simulink model "Digitizing_3delays_1us_wNodes"  (R2014a)
settings: Solver=FixedStepDiscrete  StartTime=0.0  StopTime=0.0  FixedStep=1  RelTol=1e-3
undefined symbols (not defined in the file): inputPulse
libraries: opticalComponentLibrary x22
settings Model: Creator=Nithya Menon  LastModifiedBy=Alexander

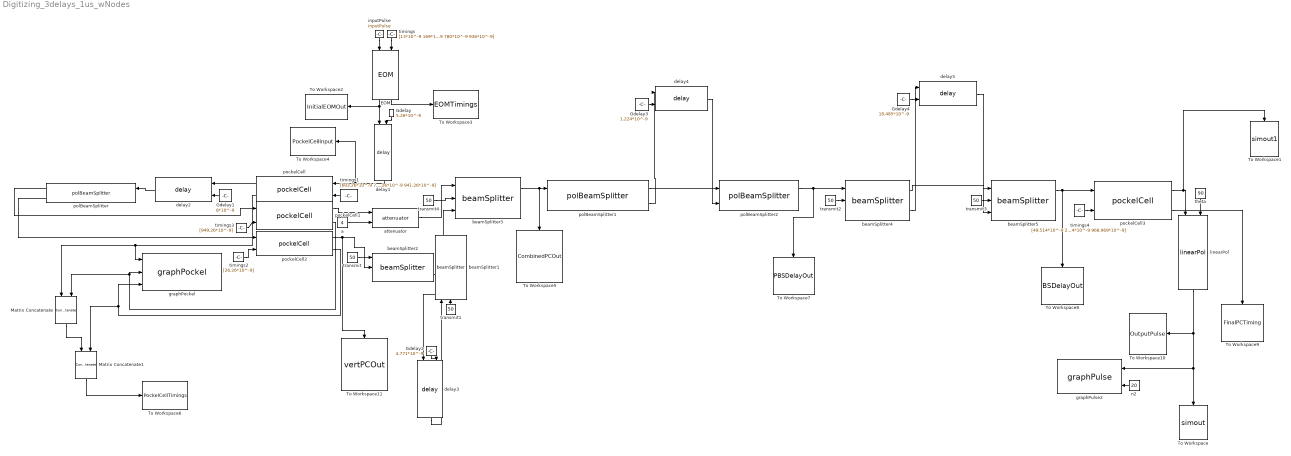
== system Digitizing_3delays_1us_wNodes ==
  EOM : opticalComponentLibrary/EOM
  Gdelay : Constant  Value=5.26*10^-9
  Gdelay1 : Constant  Value=8*10^-9
  Gdelay2 : Constant  Value=4.771*10^-9
  Gdelay3 : Constant  Value=1.224*10^-9
  Gdelay4 : Constant  Value=18.485*10^-9
  Matrix Concatenate : Concatenate  Mode=Multidimensional array  ConcatenateDimension=2
  Matrix Concatenate1 : Concatenate  Mode=Multidimensional array  ConcatenateDimension=2
  To Workspace : ToWorkspace  VariableName=simout  SampleTime=-1
  To Workspace1 : ToWorkspace  VariableName=simout1  SampleTime=-1
  To Workspace10 : ToWorkspace  VariableName=OutputPulse  SampleTime=-1
  To Workspace11 : ToWorkspace  VariableName=vertPCOut  SampleTime=-1
  To Workspace2 : ToWorkspace  VariableName=InitialEOMOut  SampleTime=-1
  To Workspace3 : ToWorkspace  VariableName=EOMTimings  SampleTime=-1
  To Workspace4 : ToWorkspace  VariableName=PockelCellInput  SampleTime=-1
  To Workspace5 : ToWorkspace  VariableName=CombinedPCOut  SampleTime=-1
  To Workspace6 : ToWorkspace  VariableName=PockelCellTimings  SampleTime=-1
  To Workspace7 : ToWorkspace  VariableName=PBSDelayOut  SampleTime=-1
  To Workspace8 : ToWorkspace  VariableName=BSDelayOut  SampleTime=-1
  To Workspace9 : ToWorkspace  VariableName=FinalPCTiming  SampleTime=-1
  a : Constant  Value=4
  attenuator : opticalComponentLibrary/attenuator
  beamSplitter{1..5} (5 alike) : opticalComponentLibrary/beamSplitter
  delay{1..5} (5 alike) : opticalComponentLibrary/delay
  graphPockel : opticalComponentLibrary/graphPockel
  graphPulse2 : opticalComponentLibrary/graphPulse
  inputPulse : Constant  Value=inputPulse
  linearPol : opticalComponentLibrary/linearPol
  n2 : Constant  Value=20
  pockelCell{,1..3} (4 alike) : opticalComponentLibrary/pockelCell
  polBeamSplitter : opticalComponentLibrary/polBeamSplitter
  polBeamSplitter1 : opticalComponentLibrary/polBeamSplitter
  polBeamSplitter2 : opticalComponentLibrary/polBeamSplitter
  theta : Constant  Value=90
  timings : Constant  Value="[13*10^-9 169*10^-9 351*10^-9  598*10^-9 780*10^-9 936*10^-9]"
  timings1 : Constant  Value=[603.26*10^-9 783.26*10^-9 941.26*10^-9]
  timings2 : Constant  Value=[26.26*10^-9]
  timings3 : Constant  Value=[949.26*10^-9]
  timings4 : Constant  Value=[49.514*10^-9 206.739*10^-9 370.254*10^-9 611.26*10^-9 811.744*10^-9 968.969*10^-9]
  transmit{,1..4} (5 alike) : Constant  Value=50
  wires:
  inputPulse/1 -> EOM/1
  timings/1 -> EOM/2
  EOM/1 -> delay1/1, To Workspace2/1
  Gdelay/1 -> delay1/2
  pockelCell/1 -> delay2/1
  Gdelay1/1 -> delay2/2
  delay2/1 -> polBeamSplitter/1
  polBeamSplitter/1 -> pockelCell1/1
  polBeamSplitter/2 -> pockelCell2/1
  pockelCell2/1 -> beamSplitter2/1, To Workspace11/1
  beamSplitter2/2 -> delay3/1
  delay3/1 -> beamSplitter1/1
  Gdelay2/1 -> delay3/2
  transmit/1 -> beamSplitter2/2
  transmit1/1 -> beamSplitter1/2
  timings1/1 -> pockelCell/2
  timings2/1 -> pockelCell2/2
  timings3/1 -> pockelCell1/2
  beamSplitter3/1 -> polBeamSplitter1/1, To Workspace5/1
  polBeamSplitter1/1 -> polBeamSplitter2/1
  polBeamSplitter1/2 -> delay4/1
  Gdelay3/1 -> delay4/2
  delay4/1 -> polBeamSplitter2/2
  transmit2/1 -> beamSplitter4/2
  transmit3/1 -> beamSplitter5/2
  beamSplitter4/1 -> beamSplitter5/1
  Gdelay4/1 -> delay5/2
  beamSplitter4/2 -> delay5/1
  delay5/1 -> beamSplitter5/3
  beamSplitter5/1 -> pockelCell3/1, To Workspace8/1
  timings4/1 -> pockelCell3/2
  pockelCell3/1 -> To Workspace1/1, linearPol/1
  delay1/1 -> To Workspace4/1, pockelCell/1
  transmit4/1 -> beamSplitter3/2
  beamSplitter1/1 -> beamSplitter3/3
  pockelCell1/1 -> attenuator/1
  attenuator/1 -> beamSplitter3/1
  a/1 -> attenuator/2
  linearPol/1 -> To Workspace10/1, graphPulse2/1, To Workspace/1
  theta/1 -> linearPol/2
  n2/1 -> graphPulse2/2
  pockelCell/2 -> Matrix Concatenate/1, graphPockel/1
  pockelCell1/2 -> Matrix Concatenate/2, graphPockel/2
  pockelCell2/2 -> Matrix Concatenate1/2, graphPockel/3
  EOM/2 -> To Workspace3/1
  Matrix Concatenate/1 -> Matrix Concatenate1/1
  Matrix Concatenate1/1 -> To Workspace6/1
  polBeamSplitter2/1 -> To Workspace7/1, beamSplitter4/1
  pockelCell3/2 -> To Workspace9/1
